simulink model "PIDDD"  (R2021a)
settings: Solver=FixedStepAuto  StartTime=0.0  StopTime=inf  FixedStep=0.002  RelTol=1e-3  EnableMultiTasking=on
libraries: arduinolib x5, dspstat3 x1, pid_lib x1
settings Model: SimulationMode=external  SILPILModeSetting=veronly  ExtModeTrigDuration=2  Creator=Juan Diego Cuesta  LastModifiedBy=Juan Diego Cuesta
settings SolverCC: AlgebraicLoopSolver=TrustRegion
settings DataIOCC: ReturnWorkspaceOutputs=off
settings OptimizationCC: PassReuseOutputArgsAs=Individual arguments  MaxStackSize=64  EfficientTunableParamExpr=on
settings DebuggingCC: ParameterTunabilityLossMsg=error  SFMachineParentedDataDiag=warning  ArithmeticOperatorsInVariantConditions=warning
settings HardwareCC: ProdBitPerPointer=32  ProdBitPerSizeT=32  ProdBitPerPtrDiffT=32  ProdLargestAtomicInteger=Long  ProdLargestAtomicFloat=Double  ProdWordSize=32  ProdHWDeviceType=ARM Compatible->ARM Cortex
settings SFSimCC: SimUseLocalCustomCode=off  MATLABDynamicMemAlloc=off  CustomCodeUndefinedFunction=UseInterfaceOnly
settings RTWCC: SystemTargetFile=ert.tlc  HardwareBoard=Arduino Due  TemplateMakefile=ert_default_tmf  GenerateReport=on  RTWUseLocalCustomCode=off  Toolchain=Arduino ARM  BuildConfiguration=Faster Runs  IncludeHyperlinkInReport=on  LaunchReport=on  GenerateTraceInfo=on  GenerateTraceReport=on  GenerateTraceReportSl=on  GenerateTraceReportSf=on  GenerateTraceReportEml=on
settings CodeAppCC: ForceParamTrailComments=on  IgnoreCustomStorageClasses=off  OperatorAnnotations=on  SimulinkDataObjDesc=on  SFDataObjDesc=on  InsertBlockDesc=on
settings ERTTargetCC: SupportContinuousTime=on  SupportVariableSizeSignals=on  ExtMode=on  ExtModeTransport=3  ExtModeStaticAlloc=on  ExtModeStaticAllocSize=24576  ExtModeMexFile=ext_xcp  ExtModeMexArgs='127.0.0.1' 0 17725  ExtModeIntrfLevel=Level2 - Open

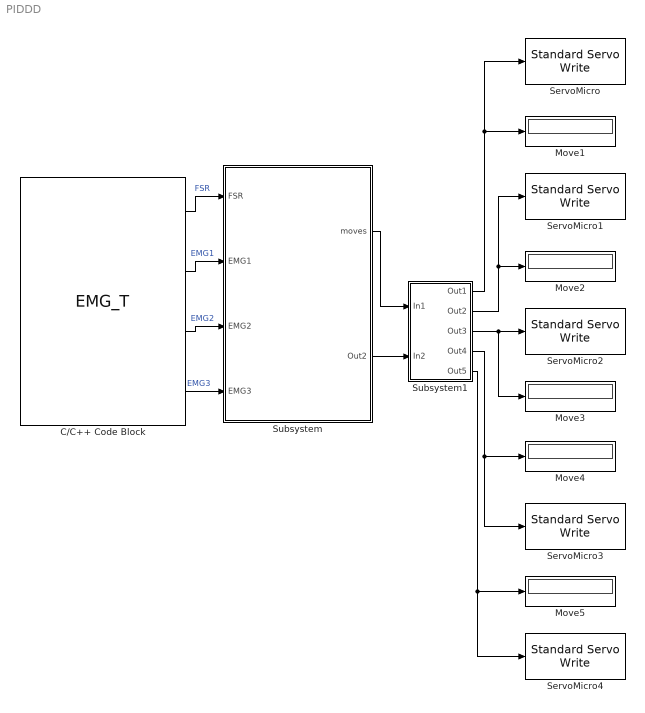
== system PIDDD ==
  C/C++ Code Block : S-Function  InitFcn=try, set_param(gcb,'FunctionName','EMG_T'), end  FunctionName=EMG_T  SFunctionModules=EMG_T_wrapper  SFunctionDeploymentMode=off  EnableBusSupport=off  mask(S-Function Builder){}
      mask help: Simulink:masks:SFunctionBuilder_MD
      mask init:
      | val = [[.9  0.75 0.75 1 1 .9 .9 1]',[1 1 0.75 0.75 .9 .9 1 .9]'];try , sys = get_param(gcb,'SfunBuilderFcnName');if isempty(sys), sys = get_param(gcb,'FunctionName'); end,catch, sys = get_param(gcb,'FunctionName'); end
      settings: CopyFcn=set_param(gcbh,'LinkStatus','none')  PreSaveFcn=try, set_param(gcb,'FunctionName','EMG_T'), end  OpenFcn=sfunctionwizard(gcbh)
      mask Display: plot(val(:,1),val(:,2)),disp(sys),port_label('output',1,'FSR'),port_label('output',2,'EMG1'),port_label('output',3,'EMG2'),port_label('output',4,'EMG3')
  Move{1..5} (5 alike) : Display
  ServoMicro : arduinolib/Standard Servo Write  pinNumber=2  ServoIndex=0  blockPlatform=arduino
  ServoMicro1 : arduinolib/Standard Servo Write  pinNumber=3  ServoIndex=1  blockPlatform=arduino
  ServoMicro2 : arduinolib/Standard Servo Write  pinNumber=4  ServoIndex=2  blockPlatform=arduino
  ServoMicro3 : arduinolib/Standard Servo Write  pinNumber=5  ServoIndex=3  blockPlatform=arduino
  ServoMicro4 : arduinolib/Standard Servo Write  pinNumber=6  ServoIndex=4  blockPlatform=arduino
  Subsystem : Subsystem
  Subsystem1 : Subsystem
  wires:
  C/C++ Code Block/2 -> Subsystem/2(EMG1)  "EMG1"
  C/C++ Code Block/1 -> Subsystem/1(FSR)  "FSR"
  C/C++ Code Block/3 -> Subsystem/3(EMG2)  "EMG2"
  Subsystem1/1(Out1) -> Move1/1, ServoMicro/1
  Subsystem/2(Out2) -> Subsystem1/2(In2)
  Subsystem1/2(Out2) -> Move2/1, ServoMicro1/1
  Subsystem/1(moves) -> Subsystem1/1(In1)
  C/C++ Code Block/4 -> Subsystem/4(EMG3)  "EMG3"
  Subsystem1/3(Out3) -> Move3/1, ServoMicro2/1
  Subsystem1/4(Out4) -> Move4/1, ServoMicro3/1
  Subsystem1/5(Out5) -> Move5/1, ServoMicro4/1

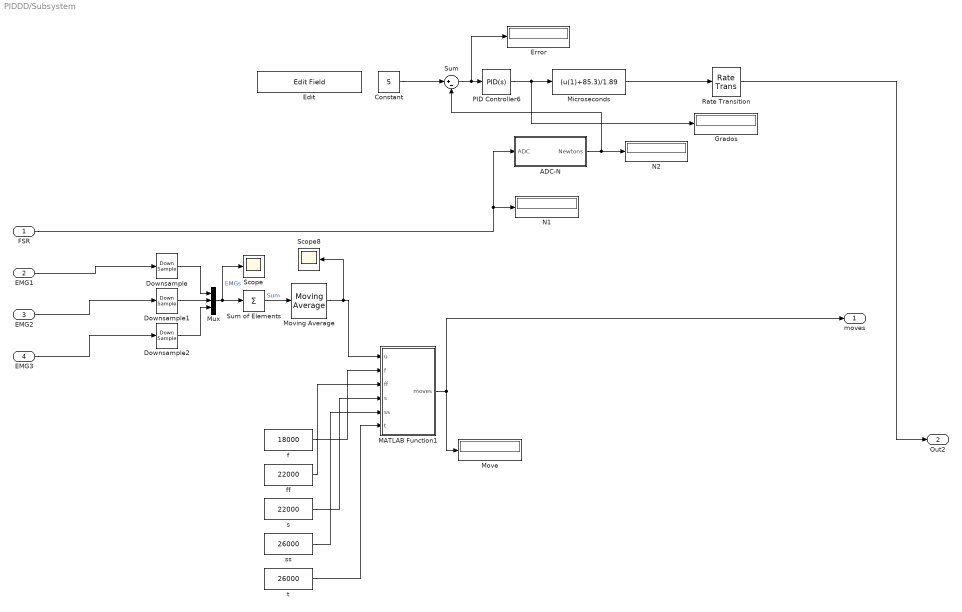
== system PIDDD/Subsystem ==
  FSR : Inport
  EMG1 : Inport  Port=2
  EMG2 : Inport  Port=3
  EMG3 : Inport  Port=4
  ADC-N : Subsystem
  Constant : Constant  Value=5
  Downsample : DownSample  N=5  RateOptions=Allow multirate processing
  Downsample1 : DownSample  N=5  RateOptions=Allow multirate processing
  Downsample2 : DownSample  N=5  RateOptions=Allow multirate processing
  Edit : EditField  LabelPosition=Hide  ShowInitialText=on  Alignment=Center
  Error : Display
  Grados : Display
  MATLAB Function1 : MATLAB Function  TreatAsAtomicUnit=on
  Microseconds : Fcn  Expr=(u(1)+85.3)/1.89
  Move : Display
  Moving Average : dspstat3/Moving Average  Method=Sliding window  ForgettingFactorPort=off  SpecifyWindowLength=on  WindowLength=200  ForgettingFactor=0.9  SimulateUsing=Code generation
  Mux : Mux  Inputs=3
  N1 : Display
  N2 : Display
  PID Controller6 : pid_lib/PID Controller  Controller=PID  Form=Ideal  TimeDomain=Continuous-time  UseExternalTs=off  SampleTime=-1  IntegratorMethod=Forward Euler  FilterMethod=Forward Euler  ControllerParametersSource=internal  P=0.245351261420682  I=13.212441112687  D=0  UseFilter=on  N=100  TunerSelectOption=Transfer Function Based (PID Tuner App)  InitialConditionSource=internal  InitialConditionForIntegrator=0  InitialConditionForFilter=0  DifferentiatorICPrevScaledInput=0  ExternalReset=none  TrackingMode=off  Kt=1  LimitOutput=on  SatLimitsSource=internal  UpperSaturationLimit=180  LowerSaturationLimit=0  LinearizeAsGain=on  AntiWindupMode=back-calculation  Kb=1  POutMin=[]  POutMax=[]  IOutMin=[]  IOutMax=[]  DOutMin=[]  DOutMax=[]  NOutMin=[]  NOutMax=[]  SumOutMin=[]  SumOutMax=[]  SaturationOutMin=[]  SaturationOutMax=[]  PParamMin=[]  PParamMax=[]  IParamMin=[]  IParamMax=[]  DParamMin=[]  DParamMax=[]  NParamMin=[]  NParamMax=[]  KbParamMin=[]  KbParamMax=[]  KtParamMin=[]  KtParamMax=[]  KbOutMin=[]  KbOutMax=[]  KtOutMin=[]  KtOutMax=[]  IntegratorOutMin=[]  IntegratorOutMax=[]  FilterOutMin=[]  FilterOutMax=[]  SumI1OutMin=[]  SumI1OutMax=[]  SumI2OutMin=[]  SumI2OutMax=[]  SumI3OutMin=[]  SumI3OutMax=[]  SumI4OutMin=[]  SumI4OutMax=[]  SumDOutMin=[]  SumDOutMax=[]  DifferentiatorOutMin=[]  DifferentiatorOutMax=[]  FilterDiffOutCoefMin=[]  FilterDiffOutCoefMax=[]  ReciprocalOutMin=[]  ReciprocalOutMax=[]  SumDenOutMin=[]  SumDenOutMax=[]  SumNumOutMin=[]  SumNumOutMax=[]  DivideOutMin=[]  DivideOutMax=[]  UdiffTsProdOutMin=[]  UdiffTsProdOutMax=[]  NTsProdOutMin=[]  NTsProdOutMax=[]  UintegralTsProdOutMin=[]  UintegralTsProdOutMax=[]  UngainTsProdOutMin=[]  UngainTsProdOutMax=[]  IntegratorContinuousStateAttributes=''  IntegratorStateMustResolveToSignalObject=off  IntegratorRTWStateStorageClass=Auto  FilterContinuousStateAttributes=''  FilterStateMustResolveToSignalObject=off  FilterRTWStateStorageClass=Auto  ParallelPVariant=Passthrough  IdealPVariant=InternalParameters  IVariant=InternalParameters  DVariant=InternalParameters  IntegratorVariant=Continuous  SatVariant=Enabled  AWVariant=BackCalculation  PCopyVariant=Disabled  TRVariant=Disabled  FdbkBlocksVariant=Forward  IdealPFdbkVariant=Disabled  SatFdbkVariant=Disabled  DerivativeFilterVariant=ContFilter  NVariant=InternalParameters  NCopyVariant=Disabled  FilterICVariant=InternalICsFilter  IntegratorICVariant=InternalICs  ExternalResetVariant=Disabled  TRSumVariant=Passthrough  SumFdbkVariant=Disabled  SumVariant=Sum_PID  TsampFilterVariant=InternalTs  TsampNgainVariant=Passthrough  TsampIntegralVariant=Passthrough  ExternalSaturationOutDataTypeStr=Inherit: Same as second input
  Rate Transition : RateTransition
  Scope : Scope
  Scope8 : Scope
  Sum : Sum  Inputs=|+-
  Sum of Elements : Sum  Inputs=+  AccumDataTypeStr=double  OutDataTypeStr=double
  f : Constant  Value=18000
  ff : Constant  Value=22000
  s : Constant  Value=22000
  ss : Constant  Value=26000
  t : Constant  Value=26000
  moves : Outport
  Out2 : Outport  Port=2
  wires:
  t/1 -> MATLAB Function1/6(t)
  Mux/1 -> Sum of Elements/1, Scope/1  "EMGs"
  Downsample/1 -> Mux/1
  Downsample2/1 -> Mux/3
  ADC-N/1(Newtons) -> Sum/2, N2/1
  EMG2/1 -> Downsample1/1
  Moving Average/1 -> MATLAB Function1/1(u), Scope8/1
  Sum of Elements/1 -> Moving Average/1  "Sum"
  Rate Transition/1 -> Out2/1
  Downsample1/1 -> Mux/2
  MATLAB Function1/1(moves) -> moves/1, Move/1
  s/1 -> MATLAB Function1/4(s)
  ss/1 -> MATLAB Function1/5(ss)
  PID Controller6/1 -> Grados/1, Microseconds/1
  Sum/1 -> PID Controller6/1, Error/1
  f/1 -> MATLAB Function1/2(f)
  FSR/1 -> ADC-N/1(ADC), N1/1
  ff/1 -> MATLAB Function1/3(ff)
  Constant/1 -> Sum/1
  Microseconds/1 -> Rate Transition/1
  EMG1/1 -> Downsample/1
  EMG3/1 -> Downsample2/1

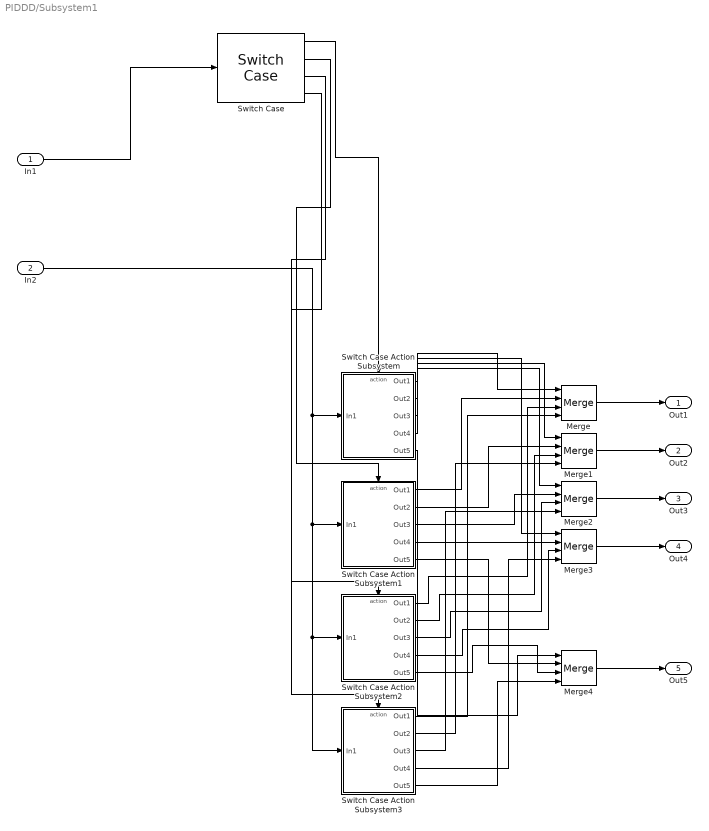
== system PIDDD/Subsystem1 ==
  In1 : Inport
  In2 : Inport  Port=2
  Merge{,1..4} (5 alike) : Merge  Inputs=4
  Switch Case : SwitchCase  CaseConditions={0,1,2,3}  ShowDefaultCase=off
  Switch Case Action Subsystem : Subsystem  TreatAsAtomicUnit=on
  Switch Case Action Subsystem1 : Subsystem  TreatAsAtomicUnit=on
  Switch Case Action Subsystem2 : Subsystem  TreatAsAtomicUnit=on
  Switch Case Action Subsystem3 : Subsystem  TreatAsAtomicUnit=on
  Out1 : Outport
  Out2 : Outport  Port=2
  Out3 : Outport  Port=3
  Out4 : Outport  Port=4
  Out5 : Outport  Port=5
  wires:
  In2/1 -> Switch Case Action Subsystem3/1(In1), Switch Case Action Subsystem2/1(In1), Switch Case Action Subsystem1/1(In1), Switch Case Action Subsystem/1(In1)
  Switch Case/4 -> Switch Case Action Subsystem2/Action
  Switch Case Action Subsystem/4(Out4) -> Merge3/1
  Switch Case Action Subsystem1/2(Out2) -> Merge1/2
  Switch Case Action Subsystem2/4(Out4) -> Merge3/3
  Switch Case Action Subsystem3/4(Out4) -> Merge3/4
  Switch Case Action Subsystem1/3(Out3) -> Merge2/2
  Merge2/1 -> Out3/1
  Switch Case/3 -> Switch Case Action Subsystem3/Action
  Switch Case Action Subsystem1/1(Out1) -> Merge/2
  Switch Case Action Subsystem2/5(Out5) -> Merge4/3
  Switch Case Action Subsystem2/2(Out2) -> Merge1/3
  Switch Case Action Subsystem/5(Out5) -> Merge4/1
  Switch Case Action Subsystem3/5(Out5) -> Merge4/4
  Switch Case Action Subsystem/3(Out3) -> Merge2/1
  Switch Case Action Subsystem1/4(Out4) -> Merge3/2
  Switch Case Action Subsystem/2(Out2) -> Merge1/1
  Switch Case Action Subsystem2/3(Out3) -> Merge2/3
  Merge4/1 -> Out5/1
  Switch Case Action Subsystem1/5(Out5) -> Merge4/2
  Merge1/1 -> Out2/1
  Switch Case Action Subsystem3/1(Out1) -> Merge/4
  Switch Case Action Subsystem2/1(Out1) -> Merge/3
  Switch Case Action Subsystem3/3(Out3) -> Merge2/4
  Switch Case/1 -> Switch Case Action Subsystem/Action
  Switch Case Action Subsystem3/2(Out2) -> Merge1/4
  In1/1 -> Switch Case/1
  Switch Case Action Subsystem/1(Out1) -> Merge/1
  Merge/1 -> Out1/1
  Switch Case/2 -> Switch Case Action Subsystem1/Action
  Merge3/1 -> Out4/1

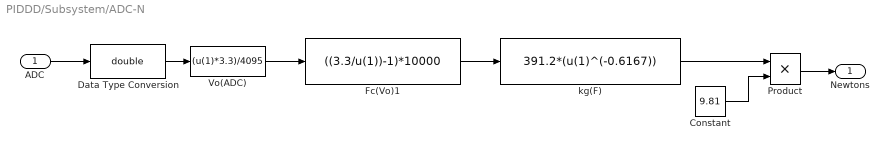
== system PIDDD/Subsystem/ADC-N ==
  ADC : Inport
  Constant : Constant  Value=9.81
  Data Type Conversion : DataTypeConversion  OutDataTypeStr=double
  Fc(Vo)1 : Fcn  Expr=((3.3/u(1))-1)*10000
  Product : Product
  Vo(ADC) : Fcn  Expr=(u(1)*3.3)/4095
  kg(F) : Fcn  Expr=391.2*(u(1)^(-0.6167))
  Newtons : Outport  VectorParamsAs1DForOutWhenUnconnected=off
  wires:
  ADC/1 -> Data Type Conversion/1
  Data Type Conversion/1 -> Vo(ADC)/1
  Vo(ADC)/1 -> Fc(Vo)1/1
  Fc(Vo)1/1 -> kg(F)/1
  kg(F)/1 -> Product/1
  Product/1 -> Newtons/1
  Constant/1 -> Product/2

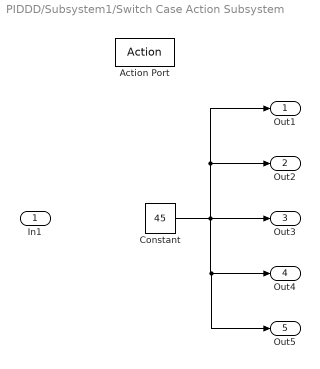
== system PIDDD/Subsystem1/Switch Case Action Subsystem ==
  In1 : Inport
  Action Port : ActionPort  ActionPortLabel=case [ 0 ]:
  Constant : Constant  Value=45  SampleTime=-1
  Out1 : Outport
  Out2 : Outport  Port=2
  Out3 : Outport  Port=3
  Out4 : Outport  Port=4
  Out5 : Outport  Port=5
  wires:
  Constant/1 -> Out3/1, Out4/1, Out5/1, Out1/1, Out2/1

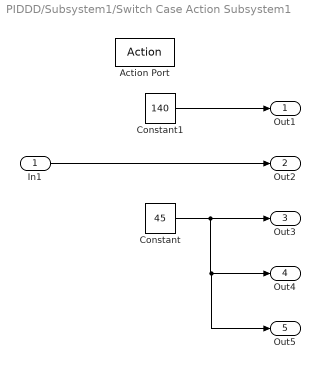
== system PIDDD/Subsystem1/Switch Case Action Subsystem1 ==
  In1 : Inport
  Action Port : ActionPort  ActionPortLabel=case [ 1 ]:
  Constant : Constant  Value=45  SampleTime=-1
  Constant1 : Constant  Value=140  SampleTime=-1
  Out1 : Outport
  Out2 : Outport  Port=2
  Out3 : Outport  Port=3
  Out4 : Outport  Port=4
  Out5 : Outport  Port=5
  wires:
  Constant/1 -> Out3/1, Out4/1, Out5/1
  In1/1 -> Out2/1
  Constant1/1 -> Out1/1

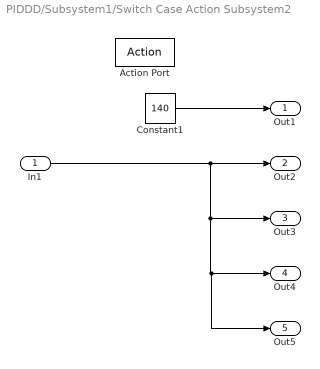
== system PIDDD/Subsystem1/Switch Case Action Subsystem2 ==
  In1 : Inport
  Action Port : ActionPort  ActionPortLabel=case [ 3 ]:
  Constant1 : Constant  Value=140  SampleTime=-1
  Out1 : Outport
  Out2 : Outport  Port=2
  Out3 : Outport  Port=3
  Out4 : Outport  Port=4
  Out5 : Outport  Port=5
  wires:
  In1/1 -> Out3/1, Out5/1, Out4/1, Out2/1
  Constant1/1 -> Out1/1

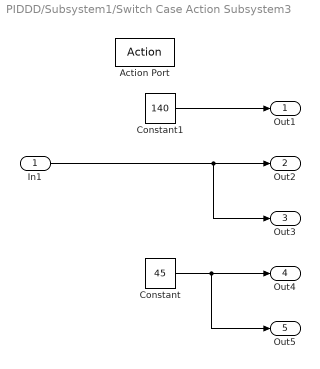
== system PIDDD/Subsystem1/Switch Case Action Subsystem3 ==
  In1 : Inport
  Action Port : ActionPort  ActionPortLabel=case [ 2 ]:
  Constant : Constant  Value=45  SampleTime=-1
  Constant1 : Constant  Value=140  SampleTime=-1
  Out1 : Outport
  Out2 : Outport  Port=2
  Out3 : Outport  Port=3
  Out4 : Outport  Port=4
  Out5 : Outport  Port=5
  wires:
  Constant/1 -> Out5/1, Out4/1
  Constant1/1 -> Out1/1
  In1/1 -> Out3/1, Out2/1

== matlab function PIDDD/Subsystem/MATLAB Function1 ==
  data: u input; moves output; f input; ff input; s input; ss input; t input
function moves = fcn(u,f,ff,s,ss,t)

if u>=f && u<=ff
    moves=1;
elseif u>=s && u<=ss
    moves=2;
elseif u>=t
    moves=3;
else
    moves=0;
end

end
